simulink model "IEEE9_16b_backward"  (R2020a)
settings: Solver=ode8  StartTime=0.0  StopTime=5  MaxStep=1e-4  RelTol=1e-3
undefined symbols (not defined in the file or in its folder): k
libraries: powerlib x33, powerlib_meascontrol x27, simulink_extras x24, dspsigops x6, sps_avr x3
(part 1 of 2)
settings Model: Creator=Pankaj  LastModifiedBy=ahmed
settings DataIOCC: ReturnWorkspaceOutputs=off
settings DebuggingCC: UnconnectedInputMsg=none  UnconnectedOutputMsg=none  UnconnectedLineMsg=none  ArithmeticOperatorsInVariantConditions=warning
settings SFSimCC: SimUseLocalCustomCode=off  CustomCodeUndefinedFunction=UseInterfaceOnly
settings RTWCC: RTWUseLocalCustomCode=off
settings CodeAppCC: StateflowObjectComments=on
settings SimscapeCC: SimscapeNormalizeSystem=off

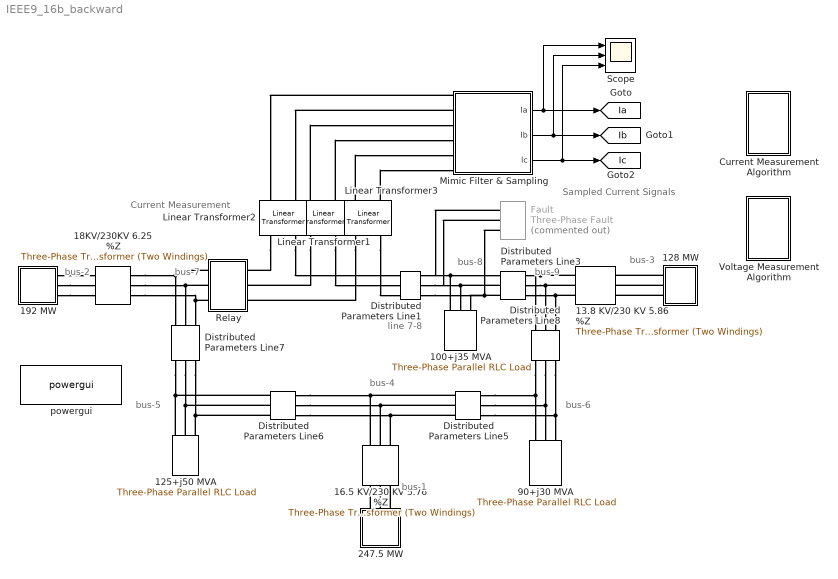
== system IEEE9_16b_backward ==
  note: bus-2
  note: bus-7
  note: bus-8
  note: bus-9
  note: bus-1
  note: bus-3
  note: bus-4
  note: bus-6
  note: bus-5
  note: line 7-8
  note: Sampled Current Signals
  note: Current Measurement
  100+j35 MVA : powerlib/Elements/Three-Phase Parallel RLC Load  LConnTagsString=A|B|C  Configuration=Y (grounded)  NominalVoltage=(230000)*0.993698  Vabc=[1e3 1e3 1e3]  Vabcp=[1e3 1e3 1e3]  NominalFrequency=60  UnbalancedPower=off  ActivePower=100e6  InductivePower=35e6  CapacitivePower=0  Pabc=[10e3 9e3 11e3]  QLabc=[100 90 110]  QCabc=[100 90 110]  Pabcp=[10e3 9e3 11e3]  QLabcp=[100 90 110]  QCabcp=[100 90 110]  Measurements=None  LoadType=constant PQ
  125+j50 MVA : powerlib/Elements/Three-Phase Parallel RLC Load  LConnTagsString=A|B|C  Configuration=Y (grounded)  NominalVoltage=(223027)*1  Vabc=[1e3 1e3 1e3]  Vabcp=[1e3 1e3 1e3]  NominalFrequency=60  UnbalancedPower=off  ActivePower=125e6  InductivePower=50e6  CapacitivePower=0  Pabc=[10e3 9e3 11e3]  QLabc=[100 90 110]  QCabc=[100 90 110]  Pabcp=[10e3 9e3 11e3]  QLabcp=[100 90 110]  QCabcp=[100 90 110]  Measurements=None  LoadType=constant PQ
  128 MW : Subsystem
  13.8 KV/230 KV 5.86 %Z : powerlib/Elements/Three-Phase Transformer (Two Windings)  Winding1Connection=Yg  Winding2Connection=Yg  CoreType=Three single-phase transformers  SetSaturation=off  Hysteresis=off  DataFile='hysteresis'  SetInitialFlux=off  Measurements=None  UNITS=pu  NominalPower=[ 100e6 , 60 ]  Winding1=[13.8e3 , 1e-6 , 0 ]  Winding2=[ 230e3 , 1e-6, 0.0586 ]  Rm=500  Lm=500  L0=0.5  Saturation=[ 0,0 ; 0.0024,1.2 ; 1.0,1.52 ]  InitialFluxes=[ 0.8 , -0.8 , 0.7 ]  BreakLoop=off  DiscreteSolver=Trapezoidal iterative  DataType=off  TransfoNumber=1
  "16.5 KV/230 KV 5.76 %Z     " : powerlib/Elements/Three-Phase Transformer (Two Windings)  Winding1Connection=Yg  Winding2Connection=Yg  CoreType=Three single-phase transformers  SetSaturation=off  Hysteresis=off  DataFile='hysteresis'  SetInitialFlux=off  Measurements=None  UNITS=pu  NominalPower=[ 100e6 , 60 ]  Winding1=[16.5e3 , 1e-6, 0 ]  Winding2=[ 230e3 ,1e-6, 0.0576 ]  Rm=500  Lm=500  L0=0.5  Saturation=[ 0,0 ; 0.0024,1.2 ; 1.0,1.52 ]  InitialFluxes=[ 0.8 , -0.8 , 0.7 ]  BreakLoop=off  DiscreteSolver=Trapezoidal iterative  DataType=off  TransfoNumber=1
  18KV/230KV 6.25 %Z : powerlib/Elements/Three-Phase Transformer (Two Windings)  Winding1Connection=Yg  Winding2Connection=Yg  CoreType=Three single-phase transformers  SetSaturation=off  Hysteresis=off  DataFile='hysteresis'  SetInitialFlux=off  Measurements=None  UNITS=pu  NominalPower=[ 100e6 , 60 ]  Winding1=[ 18e3 , 1e-6 , 0]  Winding2=[ 230e3 , 1e-6, 0.0625 ]  Rm=500  Lm=500  L0=0.5  Saturation=[ 0,0 ; 0.0024,1.2 ; 1.0,1.52 ]  InitialFluxes=[ 0.8 , -0.8 , 0.7 ]  BreakLoop=off  DiscreteSolver=Trapezoidal iterative  DataType=off  TransfoNumber=1
  192 MW : Subsystem
  247.5 MW : Subsystem
  90+j30 MVA : powerlib/Elements/Three-Phase Parallel RLC Load  LConnTagsString=A|B|C  Configuration=Y (grounded)  NominalVoltage=(226177)*0.999999  Vabc=[1e3 1e3 1e3]  Vabcp=[1e3 1e3 1e3]  NominalFrequency=60  UnbalancedPower=off  ActivePower=90e6  InductivePower=30e6  CapacitivePower=0  Pabc=[10e3 9e3 11e3]  QLabc=[100 90 110]  QCabc=[100 90 110]  Pabcp=[10e3 9e3 11e3]  QLabcp=[100 90 110]  QCabcp=[100 90 110]  Measurements=None  LoadType=constant PQ
  "Current Measurement Algorithm " : Subsystem
  Distributed Parameters Line1 : powerlib/Elements/Distributed Parameters Line  Phases=3  Frequency=60  Resistance=[0.044965 0.11241]  Inductance="[1.01e-3  2.02e-3]"  Capacitance=[12.74e-9 7.751e-9]  Length=100  x1=[-0.000416666666666667 -1.42846112004925e-12 0 0;-0.000388888888888889 -3.28216007877254e-12 0 0;-0.000361111111111111 -5.1354991116566e-12 74832.2159313653 -218040.853947513;-0.000333333333333333 -6.98827497919126e-12 77111.3845205349 -217245.270423165;-0.000305555555555556 -8.84028450362375e-12 79382.0969774256 -216425.863506783;-0.000277777777777778 -1.06913245912395e-11 81644.1042928277 -215582.72305557;-0.00025 -1.25411922546335e-11 83897.1584121488 -214715.941529378;-0.000222222222222222 -1.43896846349704e-11 86141.0122626149 -213825.613980568;-0.000194444444444444 -1.623659902423e-11 88375.4197803653 -212911.838043589;-0.000166666666666667 -1.80817328874369e-11 90600.1359374365 -211974.713924271;-0.000138888888888889 -1.99248838848699e-11 92814.9167686313 -211014.344388833;-0.000111111111111111 -2.1765849894252e-11 95019.5193982734 -210030.834752617;-8.33333333333333e-05 -2.36044290329144e-11 97213.7020668409 -209024.292868539;-5.55555555555556e-05 -2.54404196799355e-11 99397.2241574779 -207994.829115257;-2.77777777777778e-05 -2.72736204982513e-11 101569.846222381 -206942.556385074]  x2=[-0.000416666666666667 1.38170246752703e-10 0 0;-0.000388888888888889 1.35846149380387e-10 0 0;-0.000361111111111111 1.33507154946945e-10 64753.7939945472 -219178.532090877;-0.000333333333333333 1.31153519949474e-10 67045.428553326 -218488.426016288;-0.000305555555555556 1.28785502490574e-10 69329.7108253306 -217774.360223645;-0.000277777777777778 1.26403362250046e-10 71606.3903132684 -217036.41301831;-0.00025 1.2400736045641e-10 73875.2173535777 -216274.665324509;-0.000222222222222222 1.21597759858265e-10 76135.9431438061 -215489.200676461;-0.000194444444444444 1.19174824695469e-10 78388.3197698947 -214680.105209217;-0.000166666666666667 1.16738820670166e-10 80632.1002333644 -213847.467649211;-0.000138888888888889 1.14290014917651e-10 82867.0384784024 -212991.379304536;-0.000111111111111111 1.11828675977068e-10 85092.8894188446 -212111.934054926;-8.33333333333333e-05 1.0935507376197e-10 87309.4089650523 -211209.228341462;-5.55555555555556e-05 1.06869479530714e-10 89516.3540506794 -210283.361155998;-2.77777777777778e-05 1.04372165856718e-10 91713.4826593272 -209334.434030306]  x3=[-0.000416666666666667 7.37870697080606e-13 0 0;-0.000388888888888889 7.56787217936021e-13 0 0;-0.000361111111111111 7.75620748544772e-13 150.699195004272 -526.687623254678;-0.000333333333333333 7.94369223597995e-13 156.206292443821 -525.080657883959;-0.000305555555555556 8.13030587114122e-13 161.696260103119 -523.416111501981;-0.000277777777777778 8.31602792664349e-13 167.168495945345 -521.694166645014;-0.00025 8.5008380359705e-13 172.622399878173 -519.915012143715;-0.000222222222222222 8.68471593261113e-13 178.057373819577 -518.078843102425;-0.000194444444444444 8.86764145228189e-13 183.472821763418 -516.185860877771;-0.000166666666666667 9.04959453513817e-13 188.868149844801 -514.236273056586;-0.000138888888888889 9.23055522797401e-13 194.242766405203 -512.230293433144;-0.000111111111111111 9.4105036864102e-13 199.596082057352 -510.168141985716;-8.33333333333333e-05 9.58942017707044e-13 204.92750974986 -508.050044852447;-5.55555555555556e-05 9.76728507974532e-13 210.2364648316 -505.876234306557;-2.77777777777778e-05 9.94407888954391e-13 215.522365115822 -503.646948730867]  x4=[-0.000416666666666667 -1.55120252294533e-13 0 0;-0.000388888888888889 -1.82490343660272e-13 0 0;-0.000361111111111111 -2.0984042290335e-13 234.827870504209 -1040.94168030845;-0.000333333333333333 -2.37167490779369e-13 245.715473438557 -1038.42553073046;-0.000305555555555556 -2.64468550567391e-13 256.576130902281 -1035.79550609105;-0.000277777777777778 -2.91740608398552e-13 267.408651901901 -1033.05189480203;-0.00025 -3.18980673584385e-13 278.211848529418 -1030.19499773131;-0.000222222222222222 -3.46185758944774e-13 288.984536092582 -1027.22512816985;-0.000194444444444444 -3.73352881135536e-13 299.725533244803 -1024.14261179731;-0.000166666666666667 -4.00479060975577e-13 310.433662114704 -1020.94778664635;-0.000138888888888889 -4.27561323773593e-13 321.107748435285 -1017.64100306555;-0.000111111111111111 -4.54596699654279e-13 331.746621672695 -1014.22262368099;-8.33333333333333e-05 -4.81582223884008e-13 342.349115154593 -1010.69302335649;-5.55555555555556e-05 -5.08514937195951e-13 352.914066198091 -1007.05258915251;-2.77777777777778e-05 -5.35391886114587e-13 363.44031623725 -1003.30172028367]  x5=0.000395689524753941  V1=[5.416e-10 2.305e+05 2.305e+05;377 377 377;2.885 0.3359 -1.235]  V2=[2.789e-10 2.285e+05 2.285e+05;377 377 377;2.728 0.2916 -1.279]  I1=[3.179e-12 542 542;377 377 377;-1.76 0.2811 -1.29]  I2=[4.124e-12 1072 1072;377 377 377;1.614 0.2282 -1.343]  nHarmo=1  Measurements=None
  Distributed Parameters Line3 : powerlib/Elements/Distributed Parameters Line  Phases=3  Frequency=60  Resistance=[ 0.062951 0.15737]  Inductance="[ 1.414e-3  3.53e-3]"  Capacitance=[12.74e-9 7.751e-9]  Length=100  x1=[-0.000527777777777778 1.44436300590001e-10 0 0;-0.0005 1.42323859198653e-10 0 0;-0.000472222222222222 1.40195810392299e-10 0 0;-0.000444444444444444 1.38052387535472e-10 57837.2934989737 -221104.348414016;-0.000416666666666667 1.35893825678643e-10 60149.4740095849 -220486.565010016;-0.000388888888888889 1.33720361532444e-10 62455.0584525479 -219844.602769505;-0.000361111111111111 1.31532233441712e-10 64753.7939945472 -219178.532090877;-0.000333333333333333 1.29329681359349e-10 67045.428553326 -218488.426016288;-0.000305555555555556 1.27112946820012e-10 69329.7108253306 -217774.360223645;-0.000277777777777778 1.24882272913623e-10 71606.3903132684 -217036.41301831;-0.00025 1.22637904258715e-10 73875.2173535777 -216274.665324509;-0.000222222222222222 1.203800869756e-10 76135.9431438061 -215489.200676461;-0.000194444444444444 1.18109068659389e-10 78388.3197698947 -214680.105209217;-0.000166666666666667 1.15825098352831e-10 80632.1002333644 -213847.467649211;-0.000138888888888889 1.13528426519008e-10 82867.0384784024 -212991.379304536;-0.000111111111111111 1.11219305013868e-10 85092.8894188446 -212111.934054926;-8.33333333333333e-05 1.08897987058606e-10 87309.4089650523 -211209.228341462;-5.55555555555556e-05 1.06564727211894e-10 89516.3540506794 -210283.361155998;-2.77777777777778e-05 1.04219781341968e-10 91713.4826593272 -209334.434030306]  x2=[-0.000527777777777778 -2.56650173336924e-10 0 0;-0.0005 -2.57955270221522e-10 0 0;-0.000472222222222222 -2.59232079403849e-10 0 0;-0.000444444444444444 -2.60480460867389e-10 67182.8367616235 -221300.437578927;-0.000416666666666667 -2.61700277713047e-10 69496.5579996618 -220584.779459335;-0.000388888888888889 -2.6289139617416e-10 71802.6581569603 -219844.931732912;-0.000361111111111111 -2.64053685631165e-10 74100.8843436495 -219080.975532297;-0.000333333333333333 -2.65187018625927e-10 76390.9845333293 -218292.994633896;-0.000305555555555556 -2.6629127087571e-10 78672.707590707 -217481.075448696;-0.000277777777777778 -2.67366321286811e-10 80945.8032991364 -216645.307012783;-0.00025 -2.68412051967839e-10 83210.0223880579 -215785.780977586;-0.000222222222222222 -2.6942834824264e-10 85465.1165603327 -214902.59159982;-0.000194444444444444 -2.70415098662874e-10 87710.8385194724 -213995.835731153;-0.000166666666666667 -2.71372195020239e-10 89946.9419967571 -213065.612807584;-0.000138888888888889 -2.72299532358334e-10 92173.181778242 -212112.024838539;-0.000111111111111111 -2.73197008984168e-10 94389.3137316475 -211135.176395686;-8.33333333333333e-05 -2.74064526479317e-10 96595.0948331315 -210135.174601464;-5.55555555555556e-05 -2.74901989710711e-10 98790.2831939392 -209112.129117338;-2.77777777777778e-05 -2.75709306841069e-10 100974.638086929 -208066.152131775]  x3=[-0.000527777777777778 -1.02528326833281e-12 0 0;-0.0005 -1.05830185512481e-12 0 0;-0.000472222222222222 -1.09120438719242e-12 0 0;-0.000444444444444444 -1.12398725640221e-12 135.047330871066 -840.563817971818;-0.000416666666666667 -1.15664686774316e-12 143.842122898912 -839.103548572359;-0.000388888888888889 -1.18917963972083e-12 152.621141017029 -837.551262012961;-0.000361111111111111 -1.22158200475017e-12 161.383422507149 -835.907128519338;-0.000333333333333333 -1.25385040954671e-12 170.128006486366 -834.171328389256;-0.000305555555555556 -1.28598131551623e-12 178.853934012503 -832.34405197276;-0.000277777777777778 -1.31797119914282e-12 187.560248189274 -830.4254996513;-0.00025 -1.34981655237523e-12 196.24599427122 -828.415881815758;-0.000222222222222222 -1.38151388301163e-12 204.910219768403 -826.315418843377;-0.000194444444444444 -1.41305971508251e-12 213.55197455086 -824.124341073592;-0.000166666666666667 -1.44445058923189e-12 222.170310952795 -821.84288878277;-0.000138888888888889 -1.47568306309669e-12 230.764283876502 -819.471312157866;-0.000111111111111111 -1.50675371168418e-12 239.332950896006 -817.009871268981;-8.33333333333333e-05 -1.53765912774761e-12 247.875372360406 -814.458836040847;-5.55555555555556e-05 -1.56839592215984e-12 256.390611496926 -811.818486223225;-2.77777777777778e-05 -1.59896072428499e-12 264.877734513635 -809.089111360225]  x4=[-0.000527777777777778 4.46984900065056e-13 0 0;-0.0005 4.78814128694593e-13 0 0;-0.000472222222222222 5.10590849959173e-13 0 0;-0.000444444444444444 5.4231157918322e-13 129.465032115206 -498.472373255812;-0.000416666666666667 5.73972837831313e-13 134.677802784351 -497.089307540418;-0.000388888888888889 6.05571153889652e-13 139.87580451474 -495.651730380765;-0.000361111111111111 6.37103062246801e-13 145.058467286906 -494.159799423388;-0.000333333333333333 6.68565105073675e-13 150.225222763474 -492.613678275329;-0.000305555555555556 6.99953832202733e-13 155.375504351482 -491.013536486196;-0.000277777777777778 7.31265801506328e-13 160.508747264515 -489.359549529568;-0.00025 7.62497579274172e-13 165.624388584641 -487.651898783753;-0.000222222222222222 7.93645740589881e-13 170.721867324142 -485.890771511899;-0.000194444444444444 8.24706869706559e-13 175.80062448703 -484.076360841457;-0.000166666666666667 8.55677560421373e-13 180.86010313035 -482.208865743004;-0.000138888888888889 8.86554416449077e-13 185.899748425254 -480.288491008422;-0.000111111111111111 9.17334051794457e-13 190.919007717843 -478.315447228442;-8.33333333333333e-05 9.48013091123643e-13 195.917330589774 -476.289950769549;-5.55555555555556e-05 9.7858817013425e-13 200.894168918618 -474.212223750253;-2.77777777777778e-05 1.00905593592432e-12 205.848976937969 -472.082494016737]  x5=0.000523077718890797  V1=[2.541e-10 2.285e+05 2.285e+05;377 377 377;2.713 0.2668 -1.304]  V2=[4.31e-10 2.313e+05 2.313e+05;377 377 377;2.564 0.3044 -1.266]  I1=[1.418e-12 846 846;377 377 377;1.513 0.1676 -1.403]  I2=[2.062e-12 520.4 520.5;377 377 377;-2.991 0.2668 -1.304]  nHarmo=1  Measurements=None
  Distributed Parameters Line5 : powerlib/Elements/Distributed Parameters Line  Phases=3  Frequency=60  Resistance=[ 0.08993 0.224825]  Inductance="[ 1.29e-3  3.22e-3]"  Capacitance=[12.74e-9 7.751e-9]  Length=100  x1=[-0.0005 1.6339228556433e-10 59547.7501774108 -221033.498618853;-0.000472222222222222 1.62546226523253e-10 61859.095044562 -220397.806757558;-0.000444444444444444 1.61682342456709e-10 64163.6563648529 -219737.945793094;-0.000416666666666667 1.6080072809932e-10 66461.1814171648 -219053.988086653;-0.000388888888888889 1.59901480130036e-10 68751.4182519848 -218346.008641903;-0.000361111111111111 1.58984697161529e-10 71034.1157190354 -217614.085096771;-0.000333333333333333 1.58050479729384e-10 73309.0234948157 -216858.297714919;-0.000305555555555556 1.5709893028107e-10 75575.8921100521 -216078.729376952;-0.000277777777777778 1.56130153164706e-10 77834.4729770558 -215275.465571324;-0.00025 1.55144254617621e-10 80084.5184169828 -214448.594384961;-0.000222222222222222 1.541413427547e-10 82325.7816869949 -213598.206493608;-0.000194444444444444 1.53121527556531e-10 84558.0170073178 -212724.39515188;-0.000166666666666667 1.52084920857343e-10 86780.9795881935 -211827.256183037;-0.000138888888888889 1.51031636332741e-10 88994.4256567247 -210906.887968478;-0.000111111111111111 1.49961789487244e-10 91198.1124836066 -209963.391436948;-8.33333333333333e-05 1.48875497641613e-10 93391.7984097453 -208996.870053475;-5.55555555555556e-05 1.47772879919992e-10 95575.2428727585 -208007.42980802;-2.77777777777778e-05 1.46654057236839e-10 97748.2064333556 -206995.179203856]  x2=[-0.0005 -3.87923468996811e-11 47856.4063146109 -221026.29638343;-0.000472222222222222 -3.91004099718463e-11 50168.3167300571 -220513.034951382;-0.000444444444444444 -3.94041852434364e-11 52474.7256242283 -219975.591780095;-0.000416666666666667 -3.97036394020698e-11 54775.3800733984 -219414.02580627;-0.000388888888888889 -3.99987396092234e-11 57070.0277848811 -218828.398611943;-0.000361111111111111 -4.0289453503834e-11 59358.4171246963 -218218.774417737;-0.000333333333333333 -4.05757492058471e-11 61640.2971451653 -217585.220075815;-0.000305555555555556 -4.08575953197126e-11 63915.4176124293 -216927.805062548;-0.000277777777777778 -4.1134960937828e-11 66183.5290338908 -216246.601470902;-0.00025 -4.14078156439277e-11 68444.3826855732 -215541.684002527;-0.000222222222222222 -4.16761295164184e-11 70697.730639396 -214813.129959567;-0.000194444444444444 -4.19398731316604e-11 72943.3257903632 -214061.019236183;-0.000166666666666667 -4.2199017567194e-11 75180.9218836609 -213285.434309791;-0.000138888888888889 -4.24535344049117e-11 77410.273541662 -212486.460232019;-0.000111111111111111 -4.27033957341741e-11 79631.1362908349 -211664.184619378;-8.33333333333333e-05 -4.29485741548706e-11 81843.2665885521 -210818.697643655;-5.55555555555556e-05 -4.31890427804247e-11 84046.4218497981 -209950.092022024;-2.77777777777778e-05 -4.34247752407415e-11 86240.3604737711 -209058.46300688]  x3=[-0.0005 -6.00638598603095e-13 88.5700854308561 -464.00957114474;-0.000472222222222222 -6.14460049847234e-13 93.4242365008934 -463.05664410991;-0.000444444444444444 -6.28214118622572e-13 98.268142550603 -462.052937695879;-0.000416666666666667 -6.41899296640473e-13 103.101272391101 -460.998561970366;-0.000388888888888889 -6.5551408316695e-13 107.923096015235 -459.893632557552;-0.000361111111111111 -6.69056985187235e-13 112.733084655708 -458.738270625398;-0.000333333333333333 -6.82526517569508e-13 117.530710843062 -457.532602872359;-0.000305555555555556 -6.95921203227754e-13 122.315448463522 -456.276761513491;-0.000277777777777778 -7.09239573283748e-13 127.086772816688 -454.970884265952;-0.00025 -7.22480167228127e-13 131.844160673077 -453.615114333897;-0.000222222222222222 -7.35641533080558e-13 136.587090331499 -452.209600392778;-0.000194444444444444 -7.4872222754896e-13 141.31504167627 -450.754496573036;-0.000166666666666667 -7.61720816187779e-13 146.027496234245 -449.249962443204;-0.000138888888888889 -7.7463587355529e-13 150.723937231678 -447.696162992403;-0.000111111111111111 -7.87465983369912e-13 155.403849650889 -446.093268612253;-8.33333333333333e-05 -8.00209738665523e-13 160.066720286744 -444.441455078185;-5.55555555555556e-05 -8.12865741945745e-13 164.712037802931 -442.740903530168;-2.77777777777778e-05 -8.25432605337198e-13 169.339292788038 -440.991800452842]  x4=[-0.0005 7.20766318323714e-13 137.00205081313 -921.530674914054;-0.000472222222222222 7.37352059816681e-13 146.64457735357 -920.045486320562;-0.000444444444444444 7.53856942347086e-13 156.271022663568 -918.459404371524;-0.000416666666666667 7.70279155968567e-13 165.880331094918 -916.772602998701;-0.000388888888888889 7.8661689980034e-13 175.471448878661 -914.98526717887;-0.000361111111111111 8.02868382224682e-13 185.043324240651 -913.097592913547;-0.000333333333333333 8.19031821083409e-13 194.59490751689 -911.109787207486;-0.000305555555555556 8.35105443873305e-13 204.125151268634 -909.022068045984;-0.000277777777777778 8.51087487940497e-13 213.63301039726 -906.834664370972;-0.00025 8.66976200673752e-13 223.11744225887 -904.547816055915;-0.000222222222222222 8.82769839696669e-13 232.577406778632 -902.1617738795;-0.000194444444444444 8.98466673058752e-13 242.011866564832 -899.676799498139;-0.000166666666666667 9.14064979425335e-13 251.419787022637 -897.093165417278;-0.000138888888888889 9.29563048266348e-13 260.800136467551 -894.411154961508;-0.000111111111111111 9.44959180043895e-13 270.151886238551 -891.631062243498;-8.33333333333333e-05 9.60251686398627e-13 279.474010810891 -888.753192131745;-5.55555555555556e-05 9.75438890334894e-13 288.765487908559 -885.777860217136;-2.77777777777778e-05 9.90519126404638e-13 298.025298616386 -882.705392778345]  x5=0.000499582025297148  V1=[3.29e-10 2.289e+05 2.289e+05;377 377 377;2.341 0.2974 -1.273]  V2=[3.35e-10 2.261e+05 2.261e+05;377 377 377;2.353 0.2487 -1.322]  I1=[9.5e-13 477.9 477.9;377 377 377;2.529 0.2254 -1.345]  I2=[6.245e-14 926.2 926.2;377 377 377;-2.223 0.1812 -1.39]  nHarmo=1  Measurements=None
  Distributed Parameters Line6 : powerlib/Elements/Distributed Parameters Line  Phases=3  Frequency=60  Resistance=[ 0.0529 0.13225]  Inductance="[ 1.192e-3  2.38e-3]"  Capacitance=[12.74e-9 7.751e-9]  Length=100  x1=[-0.000444444444444444 9.94362101389793e-11 0 0;-0.000416666666666667 9.87568579336526e-11 51585.2167329321 -216890.72329208;-0.000388888888888889 9.80666759259649e-11 53853.6160726691 -216338.640735481;-0.000361111111111111 9.73657398021509e-11 56116.1097565287 -215762.83420901;-0.000333333333333333 9.66541264277554e-11 58372.4496765824 -215163.366856342;-0.000305555555555556 9.59319138392041e-11 60622.3883997313 -214540.304415827;-0.000277777777777778 9.5199181235246e-11 62865.67919484 -213893.715213284;-0.00025 9.44560089682681e-11 65102.0760597931 -213223.670154504;-0.000222222222222222 9.37024785354844e-11 67331.3337484726 -212530.24271748;-0.000194444444444444 9.29386725699983e-11 69553.2077976514 -211813.508944344;-0.000166666666666667 9.21646748317413e-11 71767.4545538018 -211073.54743303;-0.000138888888888889 9.13805701982875e-11 73973.8311998146 -210310.439328658;-0.000111111111111111 9.0586444655546e-11 76172.0957816271 -209524.26831463;-8.33333333333333e-05 8.97823852883316e-11 78362.0072347556 -208715.120603458;-5.55555555555556e-05 8.89684802708149e-11 80543.3254107313 -207883.084927306;-2.77777777777778e-05 8.81448188568527e-11 82715.8111034349 -207028.252528262]  x2=[-0.000444444444444444 1.61682342456709e-10 0 0;-0.000416666666666667 1.6080072809932e-10 66461.1814171648 -219053.988086653;-0.000388888888888889 1.59901480130036e-10 68751.4182519848 -218346.008641903;-0.000361111111111111 1.58984697161529e-10 71034.1157190354 -217614.085096771;-0.000333333333333333 1.58050479729384e-10 73309.0234948157 -216858.297714919;-0.000305555555555556 1.5709893028107e-10 75575.8921100521 -216078.729376952;-0.000277777777777778 1.56130153164706e-10 77834.4729770558 -215275.465571324;-0.00025 1.55144254617621e-10 80084.5184169828 -214448.594384961;-0.000222222222222222 1.541413427547e-10 82325.7816869949 -213598.206493608;-0.000194444444444444 1.53121527556531e-10 84558.0170073178 -212724.39515188;-0.000166666666666667 1.52084920857343e-10 86780.9795881935 -211827.256183037;-0.000138888888888889 1.51031636332741e-10 88994.4256567247 -210906.887968478;-0.000111111111111111 1.49961789487244e-10 91198.1124836066 -209963.391436948;-8.33333333333333e-05 1.48875497641613e-10 93391.7984097453 -208996.870053475;-5.55555555555556e-05 1.47772879919992e-10 95575.2428727585 -208007.42980802;-2.77777777777778e-05 1.46654057236839e-10 97748.2064333556 -206995.179203856]  x3=[-0.000444444444444444 8.33900745547467e-13 0 0;-0.000416666666666667 8.31603596439687e-13 105.565474688062 -1042.65174652056;-0.000388888888888889 8.29215252626237e-13 116.478085327501 -1041.4891171689;-0.000361111111111111 8.26735976015929e-13 127.377922832295 -1040.21227679903;-0.000333333333333333 8.24166038489383e-13 138.263791912432 -1038.82136543088;-0.000305555555555556 8.21505721869211e-13 149.134498809694 -1037.31653559356;-0.000277777777777778 8.18755317889107e-13 159.988851428568 -1035.69795230861;-0.00025 8.15915128161862e-13 170.825659466974 -1033.96579307194;-0.000222222222222222 8.12985464146287e-13 181.643734546788 -1032.12024783433;-0.000194444444444444 8.09966647113055e-13 192.44189034417 -1030.1615189806;-0.000166666666666667 8.06859008109473e-13 203.218942719654 -1028.08982130744;-0.000138888888888889 8.03662887923176e-13 213.973709847998 -1025.90538199987;-0.000111111111111111 8.00378637044762e-13 224.705012347794 -1023.60844060625;-8.33333333333333e-05 7.97006615629348e-13 235.41167341079 -1021.1992490121;-5.55555555555556e-05 7.93547193457082e-13 246.092518930948 -1018.67807141243;-2.77777777777778e-05 7.90000749892589e-13 256.746377633194 -1016.04518428277]  x4=[-0.000444444444444444 -4.30119678124915e-13 0 0;-0.000416666666666667 -4.36972494421452e-13 171.402870657197 -392.323506293409;-0.000388888888888889 -4.43777391759743e-13 175.501791314485 -390.507096747567;-0.000361111111111111 -4.50533623906112e-13 179.58146622263 -388.647863697952;-0.000333333333333333 -4.57240449963566e-13 183.641447999304 -386.746011030419;-0.000305555555555556 -4.63897134453051e-13 187.681291421754 -384.801747304545;-0.000277777777777778 -4.70502947394097e-13 191.700553475623 -382.815285730757;-0.00025 -4.77057164384875e-13 195.698793403535 -380.786844146953;-0.000222222222222222 -4.83559066681632e-13 199.675572753426 -378.71664499461;-0.000194444444444444 -4.90007941277513e-13 203.630455426625 -376.604915294396;-0.000166666666666667 -4.96403080980745e-13 207.56300772568 -374.451886621267;-0.000138888888888889 -5.02743784492193e-13 211.472798401915 -372.257795079081;-0.000111111111111111 -5.09029356482264e-13 215.359398702723 -370.022881274701;-8.33333333333333e-05 -5.15259107667157e-13 219.222382418584 -367.74739029161;-5.55555555555556e-05 -5.21432354884452e-13 223.061325929801 -365.431571663037;-2.77777777777778e-05 -5.27548421168026e-13 226.875808252957 -363.075679344592]  x5=0.000429504132692574  V1=[5.692e-10 2.23e+05 2.23e+05;377 377 377;2.022 0.2411 -1.33]  V2=[3.29e-10 2.289e+05 2.289e+05;377 377 377;2.367 0.3033 -1.267]  I1=[3.839e-12 1053 1053;377 377 377;3.112 0.1114 -1.459]  I2=[2.337e-12 422.3 422.3;377 377 377;0.2722 0.4185 -1.152]  nHarmo=1  Measurements=None
  Distributed Parameters Line7 : powerlib/Elements/Distributed Parameters Line  Phases=3  Frequency=60  Resistance=[ 0.16928 0.4232]  Inductance="[ 2.259e-3  5.64e-3]"  Capacitance=[12.74e-9 7.751e-9]  Length=100  x1=[-0.000666666666666667 7.99019022246078e-11 30945.1048764253 -220782.761736662;-0.000638888888888889 7.90897261162073e-11 33255.3924367584 -220446.605051692;-0.000611111111111111 7.8268876928078e-11 35562.0331685565 -220086.273912271;-0.000583333333333333 7.74394446755834e-11 37864.77412267 -219701.807832768;-0.000555555555555556 7.6601520315317e-11 40163.3627776037 -219293.248974222;-0.000527777777777778 7.57551957351273e-11 42457.5470672089 -218860.642139716;-0.0005 7.49005637440418e-11 44747.0754083251 -218404.034769463;-0.000472222222222222 7.40377180620891e-11 47031.6967283691 -217923.476935609;-0.000444444444444445 7.31667533100217e-11 49311.1604928678 -217419.021336734;-0.000416666666666667 7.22877649989394e-11 51585.2167329321 -216890.72329208;-0.000388888888888889 7.14008495198159e-11 53853.6160726692 -216338.640735481;-0.000361111111111111 7.05061041329282e-11 56116.1097565287 -215762.83420901;-0.000333333333333333 6.96036269571907e-11 58372.4496765824 -215163.366856342;-0.000305555555555556 6.86935169593958e-11 60622.3883997314 -214540.304415827;-0.000277777777777778 6.77758739433606e-11 62865.67919484 -213893.715213284;-0.00025 6.6850798538983e-11 65102.0760597932 -213223.670154504;-0.000222222222222222 6.59183921912055e-11 67331.3337484727 -212530.24271748;-0.000194444444444444 6.49787571488914e-11 69553.2077976514 -211813.508944344;-0.000166666666666667 6.4031996453612e-11 71767.4545538018 -211073.54743303;-0.000138888888888889 6.30782139283464e-11 73973.8311998147 -210310.439328658;-0.000111111111111111 6.21175141660967e-11 76172.0957816271 -209524.26831463;-8.33333333333333e-05 6.11500025184179e-11 78362.0072347556 -208715.120603458;-5.55555555555556e-05 6.01757850838651e-11 80543.3254107313 -207883.084927306;-2.77777777777778e-05 5.91949686963584e-11 82715.8111034349 -207028.252528262]  x2=[-0.000666666666666667 1.66660302751208e-11 51310.1511946695 -224554.346438586;-0.000638888888888889 1.53726448408023e-11 53658.8173143219 -224004.724189372;-0.000611111111111111 1.4077573622743e-11 56001.5991399758 -223430.537297847;-0.000583333333333333 1.27809586400961e-11 58338.2397592034 -222831.848730073;-0.000555555555555556 1.14829420813061e-11 60668.4829330292 -222208.724139;-0.000527777777777778 1.01836662885158e-11 62992.0731240297 -221561.23185726;-0.0005 8.88327374195753e-12 65308.755524356 -220889.442889679;-0.000472222222222222 7.58190704432805e-12 67618.2760836762 -220193.430905487;-0.000444444444444445 6.27970890515083e-12 69920.3815370353 -219473.272230242;-0.000416666666666667 4.97682212512627e-12 72214.8194326276 -218729.045837458;-0.000388888888888889 3.673389580472e-12 74501.3381594822 -217960.833339945;-0.000361111111111111 2.3695542072549e-12 76779.6869750537 -217168.718980862;-0.000333333333333333 1.06545898571651e-12 79049.6160327201 -216352.789624473;-0.000305555555555556 -2.38753075406283e-13 81310.8764091802 -215513.134746627;-0.000277777777777778 -1.54293895456385e-12 83563.2201317518 -214649.846424944;-0.00025 -2.84695563307772e-12 85806.400205564 -213763.019328717;-0.000222222222222222 -4.15066011082414e-12 88040.1706406435 -212852.750708531;-0.000194444444444444 -5.45390942191572e-12 90264.2864788896 -211919.140385596;-0.000166666666666667 -6.75656065037922e-12 92478.5038209373 -210962.290740807;-0.000138888888888889 -8.05847094582789e-12 94682.579852903 -209982.306703509;-0.000111111111111111 -9.35949753912663e-12 96876.2728730122 -208979.295739995;-8.33333333333333e-05 -1.06594977580483e-11 99059.3423181044 -207953.367841721;-5.55555555555556e-05 -1.19583290429191e-11 101231.548790014 -206904.635513241;-2.77777777777778e-05 -1.32558489622522e-11 103392.654081823 -205833.213759875]  x3=[-0.000666666666666667 2.48764755478526e-13 21.8432876915845 -751.401346709942;-0.000638888888888889 2.4327507735356e-13 29.7105862692523 -751.131408098936;-0.000611111111111111 2.37758721374901e-13 37.5746267463278 -750.779099464549;-0.000583333333333333 2.32216292473146e-13 45.434546742153 -750.344459441395;-0.000555555555555556 2.26648398438081e-13 53.2894843279271 -749.827535692649;-0.000527777777777778 2.21055649852032e-13 61.1385781212267 -749.228384904827;-0.0005 2.15438660022906e-13 68.9809673804663 -748.547072781563;-0.000472222222222222 2.09798044916936e-13 76.8157920992876 -747.78367403641;-0.000444444444444445 2.04134423091132e-13 84.64219310087 -746.938272384643;-0.000416666666666667 1.9844841562545e-13 92.4593121321481 -746.010960534079;-0.000388888888888889 1.92740646054684e-13 100.266291957929 -745.001840174914;-0.000361111111111111 1.87011740300088e-13 108.062276454899 -743.911021968565;-0.000333333333333333 1.81262326600738e-13 115.846410705504 -742.738625535543;-0.000305555555555556 1.75493035444635e-13 123.617841091704 -741.484779442327;-0.000277777777777778 1.69704499499569e-13 131.375715388583 -740.149621187271;-0.00025 1.63897353543737e-13 139.119182857799 -738.733297185524;-0.000222222222222222 1.58072234396134e-13 146.847394340885 -737.235962752973;-0.000194444444444444 1.52229780846717e-13 154.559502352361 -735.657782089212;-0.000166666666666667 1.46370633586356e-13 162.254661172677 -733.998928259535;-0.000138888888888889 1.40495435136575e-13 169.932026940952 -732.259583175958;-0.000111111111111111 1.34604829779092e-13 177.590757747512 -730.439937577271;-8.33333333333333e-05 1.28699463485166e-13 185.23001372622 -728.540191008118;-5.55555555555556e-05 1.22779983844757e-13 192.84895714657 -726.560551797119;-2.77777777777778e-05 1.16847039995515e-13 200.446752505559 -724.501237034023]  x4=[-0.000666666666666667 1.92335231082786e-14 62.509287542733 -294.14315595925;-0.000638888888888889 2.07829356147344e-14 65.5860561547862 -293.472443634754;-0.000611111111111111 2.23300690380977e-14 68.6556325166944 -292.76954874968;-0.000583333333333333 2.38747537177539e-14 71.7176800148185 -292.034548384372;-0.000555555555555556 2.54168202616209e-14 74.7718628611442 -291.267523139903;-0.000527777777777778 2.69560995647248e-14 77.8178461301048 -290.468557129236;-0.0005 2.84924228277437e-14 80.8552957953098 -289.637737967996;-0.000472222222222222 3.00256215755192e-14 83.8838787661745 -288.775156764868;-0.000444444444444445 3.15555276755309e-14 86.9032629244471 -287.8809081116;-0.000416666666666667 3.30819733563345e-14 89.9131171606293 -286.955090072635;-0.000388888888888889 3.46047912259596e-14 92.9131114102861 -285.997804174353;-0.000361111111111111 3.61238142902662e-14 95.9029166902411 -285.009155393941;-0.000333333333333333 3.76388759712576e-14 98.8822051346535 -283.989252147879;-0.000305555555555556 3.91498101253471e-14 101.850650030972 -282.938206280051;-0.000277777777777778 4.0656451061578e-14 104.807925855761 -281.85613304948;-0.00025 4.21586335597936e-14 107.753708310403 -280.743151117691;-0.000222222222222222 4.36561928887547e-14 110.687674356655 -279.599382535694;-0.000194444444444444 4.51489648242049e-14 113.609502252076 -278.424952730603;-0.000166666666666667 4.66367856668796e-14 116.518871585313 -277.219990491881;-0.000138888888888889 4.81194922604571e-14 119.415463311232 -275.984627957217;-0.000111111111111111 4.95969220094509e-14 122.29895978591 -274.719000598033;-8.33333333333333e-05 5.10689128970398e-14 125.169044801462 -273.423247204631;-5.55555555555556e-05 5.25353035028352e-14 128.025403620726 -272.097509870974;-2.77777777777778e-05 5.39959330205825e-14 130.867723011767 -270.741933979099]  x5=0.000661178039562719  V1=[5.692e-10 2.23e+05 2.23e+05;377 377 377;1.934 0.1858 -1.385]  V2=[7.107e-10 2.305e+05 2.305e+05;377 377 377;2.15 0.2689 -1.302]  I1=[1.362e-12 746.7 746.7;377 377 377;1.537 0.07174 -1.499]  I2=[6.286e-13 306.4 306.4;377 377 377;-2.668 0.2582 -1.313]  nHarmo=1  Measurements=None
  Distributed Parameters Line8 : powerlib/Elements/Distributed Parameters Line  Phases=3  Frequency=60  Resistance=[ 0.20631 0.5157]  Inductance="[ 2.38e-3  6.09e-3]"  Capacitance=[12.74e-9 7.751e-9]  Length=100  x1=[-0.000694444444444444 -4.21682122231462e-11 0 0;-0.000666666666666667 -4.22842201571023e-11 0 0;-0.000638888888888889 -4.23955911498183e-11 0 0;-0.000611111111111111 -4.25023129882099e-11 0 0;-0.000583333333333333 -4.26043739690248e-11 0 0;-0.000555555555555556 -4.27017629001263e-11 43217.0956035148 -221980.051548184;-0.000527777777777778 -4.27944691017207e-11 45539.2479049196 -221515.31979134;-0.0005 -4.28824824075282e-11 47856.4063146109 -221026.29638343;-0.000472222222222222 -4.29657931658982e-11 50168.3167300571 -220513.034951382;-0.000444444444444444 -4.30443922408669e-11 52474.7256242283 -219975.591780095;-0.000416666666666667 -4.31182710131603e-11 54775.3800733984 -219414.02580627;-0.000388888888888889 -4.31874213811383e-11 57070.0277848811 -218828.398611943;-0.000361111111111111 -4.32518357616839e-11 59358.4171246963 -218218.774417737;-0.000333333333333333 -4.33115070910343e-11 61640.2971451653 -217585.220075815;-0.000305555555555556 -4.33664288255559e-11 63915.4176124293 -216927.805062548;-0.000277777777777778 -4.34165949424615e-11 66183.5290338908 -216246.601470902;-0.00025 -4.34619999404711e-11 68444.3826855732 -215541.684002527;-0.000222222222222222 -4.35026388404151e-11 70697.730639396 -214813.129959567;-0.000194444444444444 -4.353850718578e-11 72943.3257903632 -214061.019236183;-0.000166666666666667 -4.35696010431975e-11 75180.9218836609 -213285.434309791;-0.000138888888888889 -4.3595917002876e-11 77410.273541662 -212486.460232019;-0.000111111111111111 -4.36174521789737e-11 79631.1362908349 -211664.184619378;-8.33333333333333e-05 -4.3634204209916e-11 81843.2665885521 -210818.697643655;-5.55555555555556e-05 -4.36461712586539e-11 84046.4218497981 -209950.092022024;-2.77777777777778e-05 -4.36533520128656e-11 86240.3604737711 -209058.46300688]  x2=[-0.000694444444444444 -2.48233780060832e-10 0 0;-0.000666666666666667 -2.49705490214106e-10 0 0;-0.000638888888888889 -2.51149817346452e-10 0 0;-0.000611111111111111 -2.52566603071126e-10 0 0;-0.000583333333333333 -2.53955692021605e-10 0 0;-0.000555555555555556 -2.55316931868634e-10 57856.8274653565 -223919.64435805;-0.000527777777777778 -2.56650173336924e-10 60198.4878307961 -223301.502811592;-0.0005 -2.57955270221522e-10 62533.5467536697 -222658.873738972;-0.000472222222222222 -2.59232079403849e-10 64861.7481684527 -221991.827611708;-0.000444444444444444 -2.60480460867389e-10 67182.8367616235 -221300.437578927;-0.000416666666666667 -2.61700277713047e-10 69496.5579996618 -220584.779459335;-0.000388888888888889 -2.6289139617416e-10 71802.6581569603 -219844.931732912;-0.000361111111111111 -2.64053685631165e-10 74100.8843436495 -219080.975532297;-0.000333333333333333 -2.65187018625927e-10 76390.9845333293 -218292.994633896;-0.000305555555555556 -2.6629127087571e-10 78672.707590707 -217481.075448696;-0.000277777777777778 -2.67366321286811e-10 80945.8032991364 -216645.307012783;-0.00025 -2.68412051967839e-10 83210.0223880579 -215785.780977586;-0.000222222222222222 -2.6942834824264e-10 85465.1165603327 -214902.59159982;-0.000194444444444444 -2.70415098662874e-10 87710.8385194724 -213995.835731153;-0.000166666666666667 -2.71372195020239e-10 89946.9419967571 -213065.612807584;-0.000138888888888889 -2.72299532358334e-10 92173.181778242 -212112.024838539;-0.000111111111111111 -2.73197008984168e-10 94389.3137316475 -211135.176395686;-8.33333333333333e-05 -2.74064526479317e-10 96595.0948331315 -210135.174601464;-5.55555555555556e-05 -2.74901989710711e-10 98790.2831939392 -209112.129117338;-2.77777777777778e-05 -2.75709306841069e-10 100974.638086929 -208066.152131775]  x3=[-0.000694444444444444 2.67943583314178e-13 0 0;-0.000666666666666667 2.57457326892443e-13 0 0;-0.000638888888888889 2.46942837373535e-13 0 0;-0.000611111111111111 2.36401267789715e-13 0 0;-0.000583333333333333 2.25833774142883e-13 0 0;-0.000555555555555556 2.152415152778e-13 58.759105057336 -662.748688309064;-0.000527777777777778 2.04625652755016e-13 65.6960390810262 -662.09704112072;-0.0005 1.93987350723485e-13 72.6257687937041 -661.372787530662;-0.000472222222222222 1.83327775792909e-13 79.5475342724156 -660.576006961456;-0.000444444444444444 1.72648096905801e-13 86.4605764675751 -659.706786789073;-0.000416666666666667 1.619494852093e-13 93.3641372862026 -658.765222333299;-0.000388888888888889 1.51233113926741e-13 100.257459675059 -657.751416847286;-0.000361111111111111 1.40500158228998e-13 107.139787703662 -656.665481506231;-0.000333333333333333 1.29751795105612e-13 114.010366647189 -655.507535395182;-0.000305555555555556 1.18989203235723e-13 120.868443069232 -654.277705495978;-0.000277777777777778 1.08213562858812e-13 127.713264904429 -652.976126673327;-0.00025 9.74260556452786e-14 134.544081540932 -651.602941660014;-0.000222222222222222 8.66278645668514e-14 141.36014390272 -650.15830104125;-0.000194444444444444 7.58201737668671e-14 148.160704531745 -648.642363238159;-0.000166666666666667 6.50041684304136e-14 154.945017669899 -647.055294490404;-0.000138888888888889 5.41810346543613e-14 161.712339340793 -645.397268837957;-0.000111111111111111 4.33519593172943e-14 168.461927431347 -643.668468102016;-8.33333333333333e-05 3.25181299493561e-14 175.193041773164 -641.869081865064;-5.55555555555556e-05 2.16807346020229e-14 181.904944223704 -639.999307450078;-2.77777777777778e-05 1.08409617178209e-14 188.596898747228 -638.059349898893]  x4=[-0.000694444444444444 -6.35781979912706e-13 0 0;-0.000666666666666667 -6.27654481410824e-13 0 0;-0.000638888888888889 -6.19458153522031e-13 0 0;-0.000611111111111111 -6.11193895066046e-13 0 0;-0.000583333333333333 -6.02862612311938e-13 0 0;-0.000555555555555556 -5.94465218878746e-13 61.9212558415062 -356.348275740455;-0.000527777777777778 -5.86002635635289e-13 65.649444258534 -355.680308951777;-0.0005 -5.77475790599186e-13 69.370433474197 -354.97333780907;-0.000472222222222222 -5.68885618835083e-13 73.0838154400958 -354.227439839686;-0.000444444444444444 -5.60233062352116e-13 76.7891829420518 -353.442696839744;-0.000416666666666667 -5.51519070000609e-13 80.4861296447628 -352.619194865156;-0.000388888888888889 -5.42744597368022e-13 84.174250136362 -351.757024222193;-0.000361111111111111 -5.33910606674158e-13 87.8531399728761 -350.856279457584;-0.000333333333333333 -5.25018066665646e-13 91.5223957225774 -349.917059348141;-0.000305555555555556 -5.16067952509709e-13 95.181615010224 -348.939466889933;-0.000277777777777778 -5.07061245687222e-13 98.8303965611854 -347.923609286991;-0.00025 -4.97998933885084e-13 102.468340245447 -346.869597939548;-0.000222222222222222 -4.88882010887908e-13 106.095047121487 -345.777548431825;-0.000194444444444444 -4.79711476469038e-13 109.710119480027 -344.647580519359;-0.000166666666666667 -4.70488336280917e-13 113.313160887646 -343.479818115863;-0.000138888888888889 -4.612136017448e-13 116.90377623025 -342.274389279644;-0.000111111111111111 -4.51888289939848e-13 120.481571756405 -341.03142619956;-8.33333333333333e-05 -4.42513423491586e-13 124.046155120513 -339.751065180518;-5.55555555555556e-05 -4.33090030459764e-13 127.597135425839 -338.433446628532;-2.77777777777778e-05 -4.23619144225622e-13 131.134123267376 -337.078715035326]  x5=0.000687048688231045  V1=[3.258e-10 2.261e+05 2.261e+05;377 377 377;2.369 0.194 -1.377]  V2=[4.31e-10 2.313e+05 2.313e+05;377 377 377;2.502 0.2568 -1.314]  I1=[9.177e-13 670.6 670.6;377 377 377;2.076 0.09296 -1.478]  I2=[4.71e-13 356.3 356.3;377 377 377;-2.438 0.173 -1.398]  nHarmo=1  Measurements=None
  Fault : powerlib/Elements/Three-Phase Fault  Commented=on  InitialStates=0  FaultA=on  FaultB=off  FaultC=off  GroundFault=on  SwitchTimes=1  External=off  SwitchStatus=NaN  FaultResistance=1e-100  GroundResistance=0.01  SnubberResistance=1e6  SnubberCapacitance=inf  Measurements=None
  Linear Transformer1 : powerlib/Elements/Linear Transformer  UNITS=pu  NominalPower=[ 150e8 60 ]  winding1=[230e3 0.002 1]  winding2=[230e3 0.002 1]  ThreeWindings=off  winding3=[3.15e+05 0.002 0.079997]  RmLm=[499.99 500]  Measurements=None  DataType=off
  Linear Transformer2 : powerlib/Elements/Linear Transformer  UNITS=pu  NominalPower=[ 150e8 60 ]  winding1=[230e3 0.002 1]  winding2=[230e3 0.002 1]  ThreeWindings=off  winding3=[3.15e+05 0.002 0.079997]  RmLm=[499.99 500]  Measurements=None  DataType=off
  Linear Transformer3 : powerlib/Elements/Linear Transformer  UNITS=pu  NominalPower=[ 150e8 60 ]  winding1=[230e3 0.002 1]  winding2=[230e3 0.002 1]  ThreeWindings=off  winding3=[3.15e+05 0.002 0.079997]  RmLm=[499.99 500]  Measurements=None  DataType=off
  Mimic Filter & Sampling : Subsystem
  Relay : Subsystem
  Scope : Scope  NumInputPorts=3
  Voltage Measurement Algorithm : Subsystem
  powergui : powerlib/powergui  Priority=1  SimulationMode=Discrete  SampleTime=1/1200/30  frequency=60  Iterations=50  frequencyindice=60  Pbase=100e6  ErrMax=0.0001  UnitsV=kV  UnitsW=MW  buscounter=0  FunctionMessages=off  echomessages=off  EnableUseOfTLC=off  CurrentSourceSwitches=off  DisableSnubberDevices=off  DisableRonSwitches=off  DisableVfSwitches=off  DisplayEquations=off  AutomaticDiscreteSolvers=off  SolverType=Tustin/Backward Euler (TBE)  Interpol=off  ExternalGateDelay=off  methode=off  Ts=100  x0status=blocks  SPID=on  SwTol=0  HookPort=off  NonlinearTolerance=1e-4  nMaxIteration=100  ContinueOnMaxIteration=off  RestoreLinks=warning  ResistiveCurrentMeasurement=off  Frange=[0:2:500]  Ylog=off  Xlog=on  ShowGrid=off  save=off  variable=ZData  structure=0  ZoomFFT=off  StartTime=0.0  cycles=1  DisplayStyle=1  fundamental=60  FreqAxis=off  MaxFrequency=1000  frequencyindicesteady=1  RmsSteady=1  display=off
  tag scope: Ia=global, Ib=global, Ic=global
  wires:
  Mimic Filter & Sampling/1(Ia) -> Scope/1, [Ia]
  Mimic Filter & Sampling/2(Ib) -> Scope/2, [Ib]
  Mimic Filter & Sampling/3(Ic) -> Scope/3, [Ic]
  connections:
  Distributed Parameters Line3/LConn2 -- Distributed Parameters Line1/RConn2 -- Fault/LConn2 -- 100+j35 MVA/LConn2
  Distributed Parameters Line3/LConn3 -- Distributed Parameters Line1/RConn3 -- 100+j35 MVA/LConn3 -- Fault/LConn3
  Distributed Parameters Line5/RConn1 -- Distributed Parameters Line8/LConn1 -- 90+j30 MVA/LConn1
  Distributed Parameters Line5/RConn3 -- Distributed Parameters Line8/LConn3 -- 90+j30 MVA/LConn3
  Distributed Parameters Line6/LConn1 -- Distributed Parameters Line7/LConn1 -- 125+j50 MVA/LConn1
  Distributed Parameters Line6/LConn2 -- Distributed Parameters Line7/LConn2 -- 125+j50 MVA/LConn2
  Distributed Parameters Line6/LConn3 -- Distributed Parameters Line7/LConn3 -- 125+j50 MVA/LConn3
  Distributed Parameters Line3/RConn1 -- Distributed Parameters Line8/RConn1 -- 13.8 KV/230 KV 5.86 %Z/RConn1
  Distributed Parameters Line3/RConn2 -- 13.8 KV/230 KV 5.86 %Z/RConn2 -- Distributed Parameters Line8/RConn2
  Distributed Parameters Line3/RConn3 -- 13.8 KV/230 KV 5.86 %Z/RConn3 -- Distributed Parameters Line8/RConn3
  18KV/230KV 6.25 %Z/RConn1 -- Relay/LConn1 -- Distributed Parameters Line7/RConn1
  18KV/230KV 6.25 %Z/RConn2 -- Relay/LConn2 -- Distributed Parameters Line7/RConn2
  18KV/230KV 6.25 %Z/RConn3 -- Relay/LConn3 -- Distributed Parameters Line7/RConn3
  Distributed Parameters Line5/RConn2 -- Distributed Parameters Line8/LConn2 -- 90+j30 MVA/LConn2
  Distributed Parameters Line6/RConn1 -- "16.5 KV/230 KV 5.76 %Z     "/RConn1 -- Distributed Parameters Line5/LConn1
  Distributed Parameters Line6/RConn2 -- "16.5 KV/230 KV 5.76 %Z     "/RConn2 -- Distributed Parameters Line5/LConn2
  Distributed Parameters Line6/RConn3 -- "16.5 KV/230 KV 5.76 %Z     "/RConn3 -- Distributed Parameters Line5/LConn3
  247.5 MW/RConn1 -- "16.5 KV/230 KV 5.76 %Z     "/LConn1
  247.5 MW/RConn2 -- "16.5 KV/230 KV 5.76 %Z     "/LConn2
  247.5 MW/RConn3 -- "16.5 KV/230 KV 5.76 %Z     "/LConn3
  128 MW/RConn1 -- 13.8 KV/230 KV 5.86 %Z/LConn1
  128 MW/RConn2 -- 13.8 KV/230 KV 5.86 %Z/LConn2
  128 MW/RConn3 -- 13.8 KV/230 KV 5.86 %Z/LConn3
  192 MW/RConn1 -- 18KV/230KV 6.25 %Z/LConn1
  192 MW/RConn2 -- 18KV/230KV 6.25 %Z/LConn2
  192 MW/RConn3 -- 18KV/230KV 6.25 %Z/LConn3
  Mimic Filter & Sampling/LConn1 -- Linear Transformer2/RConn1
  Mimic Filter & Sampling/LConn2 -- Linear Transformer2/RConn2
  Linear Transformer1/RConn1 -- Mimic Filter & Sampling/LConn3
  Linear Transformer1/RConn2 -- Mimic Filter & Sampling/LConn4
  Linear Transformer3/RConn1 -- Mimic Filter & Sampling/LConn5
  Linear Transformer3/RConn2 -- Mimic Filter & Sampling/LConn6
  100+j35 MVA/LConn1 -- Fault/LConn1 -- Distributed Parameters Line1/RConn1 -- Distributed Parameters Line3/LConn1
  Linear Transformer2/LConn1 -- Relay/RConn1
  Linear Transformer2/LConn2 -- Distributed Parameters Line1/LConn1
  Linear Transformer1/LConn1 -- Relay/RConn2
  Linear Transformer1/LConn2 -- Distributed Parameters Line1/LConn2
  Linear Transformer3/LConn1 -- Relay/RConn3
  Linear Transformer3/LConn2 -- Distributed Parameters Line1/LConn3

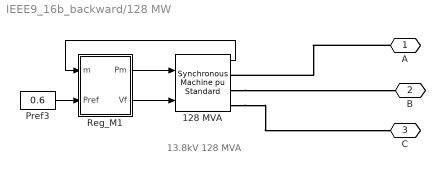
== system IEEE9_16b_backward/128 MW ==
  note: 13.8kV 128 MVA
  128 MVA : powerlib/Machines/Synchronous Machine pu Standard  PresetModel=No  MechanicalLoad=Mechanical power Pm  ShowDetailedParameters=on  RotorType=Salient-pole  Units=per unit standard parameters  MeasurementBus=off  NominalParameters="[128e6  13800   60 ]"  Reactances1=[ 31 32 33 34 35 36 37 ]  Reactances2=[ 1.305, 0.296, 0.252, 0.474, 0.243, 0.18 ]  dAxisTimeConstants=Short-circuit  qAxisTimeConstants=Open-circuit  TimeConstants1=[]  TimeConstants2=[]  TimeConstants3=[]  TimeConstants4=[]  TimeConstants5=[ 1.01, 0.053, 0.1 ]  TimeConstants6=[]  TimeConstants7=[]  TimeConstants8=[]  StatorResistance=2.8544e-3  Mechanical="[20 0  32]"  PolePairs=32  InitialConditions=[0 -74.5248 0.603223 0.603223 0.603223 5.08525 -114.915 125.085 1.10339]  SetSaturation=off  Saturation=[0.6404,0.7127,0.8441,0.9214,0.9956,1.082,1.19,1.316,1.457;0.7,0.7698,0.8872,0.9466,0.9969,1.046,1.1,1.151,1.201]  LoadFlowParameters=[1 500000000 0 0 0]  TsPowergui=0  TsBlock=-1  IterativeModel=Trapezoidal non iterative  IterativeDiscreteModel=Trapezoidal non iterative  BusType=PV  Pref=0.6*128e6  Qref=0  Qmin=-Inf  Qmax=Inf  PLF=0  QLF=0
      settings: AttributesFormatString=\n\n
  Pref3 : Constant  Value=0.6
  Reg_M1 : Subsystem
  A : PMIOPort  Side=Right
  B : PMIOPort  Port=2  Side=Right
  C : PMIOPort  Port=3  Side=Right
  wires:
  Reg_M1/1(Pm) -> 128 MVA/1
  Reg_M1/2(Vf) -> 128 MVA/2
  Pref3/1 -> Reg_M1/2(Pref)
  128 MVA/1 -> Reg_M1/1(m)
  connections:
  A/RConn1 -- 128 MVA/RConn1
  128 MVA/RConn2 -- B/RConn1
  128 MVA/RConn3 -- C/RConn1
